simulink model "Pcontroller"  (R2020a)
settings: Solver=VariableStepAuto  StartTime=0.0  StopTime=10.0  RelTol=1e-3
settings Model: Creator=Ishan's PC  LastModifiedBy=Ishan's PC

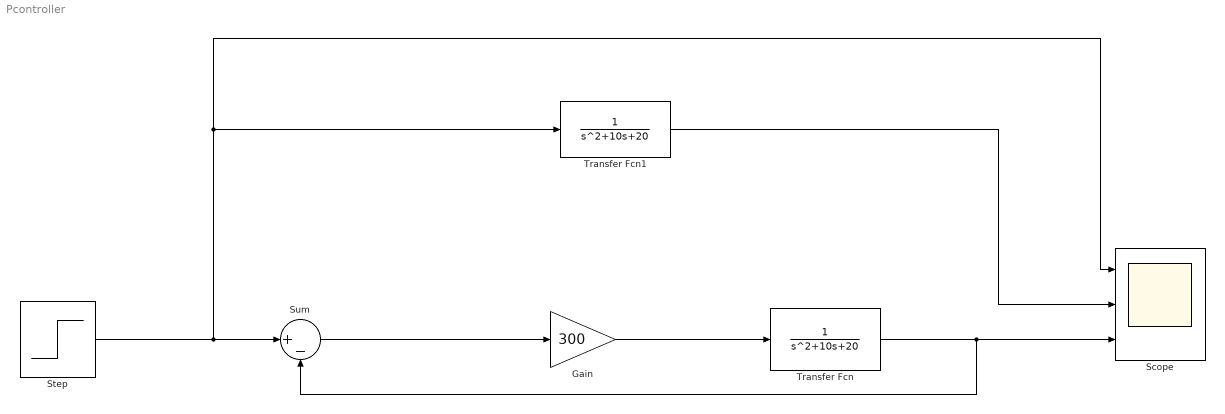
== system Pcontroller ==
  Gain : Gain  Gain=300
  Scope : Scope  NumInputPorts=3
  Step : Step  SampleTime=0
  Sum : Sum  Inputs=|+-
  Transfer Fcn : TransferFcn  Denominator=[1 10 20]
  Transfer Fcn1 : TransferFcn  Denominator=[1 10 20]
  wires:
  Sum/1 -> Gain/1
  Gain/1 -> Transfer Fcn/1
  Transfer Fcn/1 -> Sum/2, Scope/3
  Step/1 -> Transfer Fcn1/1, Scope/1, Sum/1
  Transfer Fcn1/1 -> Scope/2
